simulink model "hybridmodel_arduino"  (R2017a)
settings: Solver=VariableStepAuto  StartTime=0.0  StopTime=5  RelTol=1e-3
values from neighbouring files (symbols this model uses):
  a = 25.1133    [params.m]
  IRQ_DELAY = computation_time + delay    (= 0.00087)    [params.m]
  K = 1    [params.m]
  T = 1/Fs    (= 0.002)    [params.m]
  zg = K*(1-exp(-a*T))    [params.m]
  zp = exp(-a*T)    [params.m]
settings Model: Creator=Merc  LastModifiedBy=Merc

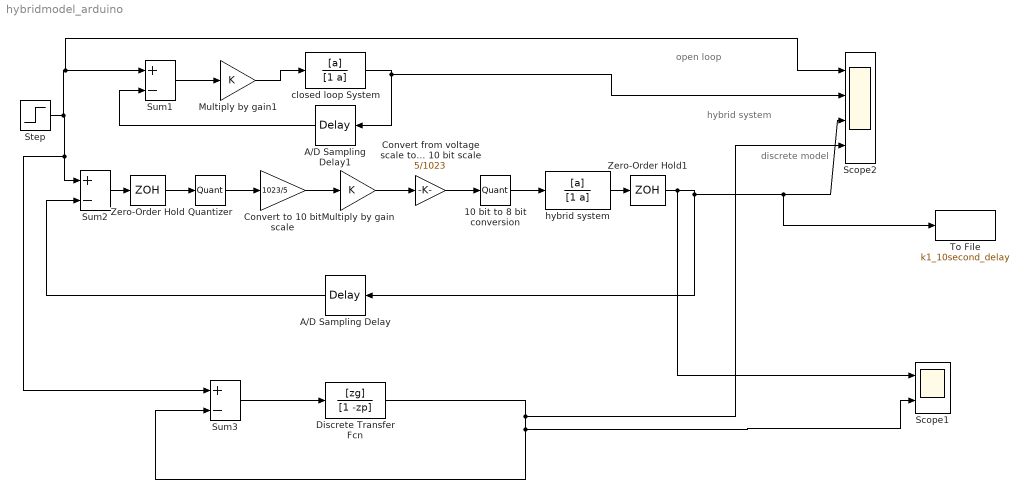
== system hybridmodel_arduino ==
  note: discrete model
  note: open loop
  note: hybrid system
  10 bit to 8 bit conversion : Quantizer  QuantizationInterval=(5/2^8)
  A/D Sampling Delay : TransportDelay  DelayTime=IRQ_DELAY
  A/D Sampling Delay1 : TransportDelay  DelayTime=IRQ_DELAY
  Convert from voltage scale to 10 bit scale : Gain  Gain=5/1023
  Convert to 10 bit scale : Gain  Gain=1023/5
  Discrete Transfer Fcn : DiscreteTransferFcn  Numerator=[zg]  Denominator=[1 -zp]  SampleTime=T
  Multiply by gain : Gain  Gain=K
  Multiply by gain1 : Gain  Gain=K
  Quantizer : Quantizer  QuantizationInterval=(5/2^10)
  Scope1 : Scope  NumInputPorts=2
  Scope2 : Scope  NumInputPorts=4
  Step : Step  SampleTime=0
  Sum1 : Sum  Inputs=+-
  Sum2 : Sum  Inputs=+-
  Sum3 : Sum  Inputs=+-
  To File : ToFile  Filename=k1_10second_delay  SaveFormat=Timeseries
  Zero-Order Hold : ZeroOrderHold  SampleTime=T
  Zero-Order Hold1 : ZeroOrderHold  SampleTime=T
  "closed loop System " : TransferFcn  Numerator=[a]  Denominator=[1 a]
  hybrid system : TransferFcn  Numerator=[a]  Denominator=[1 a]
  wires:
  Zero-Order Hold/1 -> Quantizer/1
  Quantizer/1 -> Convert to 10 bit scale/1
  Multiply by gain/1 -> Convert from voltage scale to 10 bit scale/1
  Convert from voltage scale to 10 bit scale/1 -> 10 bit to 8 bit conversion/1
  Sum2/1 -> Zero-Order Hold/1
  Step/1 -> Sum1/1, Scope2/1, Sum3/1, Sum2/1
  Sum3/1 -> Discrete Transfer Fcn/1
  Discrete Transfer Fcn/1 -> Scope2/4, Scope1/2, Sum3/2
  Sum1/1 -> Multiply by gain1/1
  Multiply by gain1/1 -> "closed loop System "/1
  "closed loop System "/1 -> Scope2/2, A/D Sampling Delay1/1
  A/D Sampling Delay1/1 -> Sum1/2
  hybrid system/1 -> Zero-Order Hold1/1
  Convert to 10 bit scale/1 -> Multiply by gain/1
  10 bit to 8 bit conversion/1 -> hybrid system/1
  Zero-Order Hold1/1 -> Scope1/1, To File/1, Scope2/3, A/D Sampling Delay/1
  A/D Sampling Delay/1 -> Sum2/2
